simulink model "wheelControl"  (R2015a)
settings: Solver=ode45  StartTime=0.0  StopTime=10.0  RelTol=1e-3
libraries: simulink x2
settings Model: Creator=julig  LastModifiedBy=julig

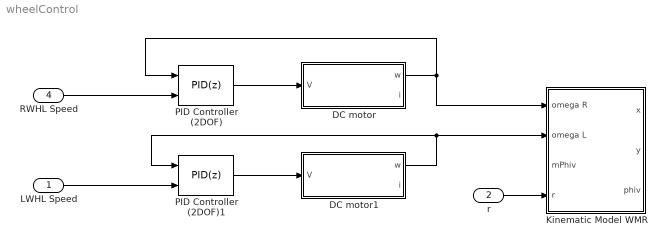
== system wheelControl ==
  "LWHL Speed " : Inport
  r : Inport  Port=2
  "RWHL Speed " : Inport  Port=4
  DC motor : Subsystem  mask(DC Motor){L=0.1, Kphi=0.3, J=0.1, b=0.01, R=2}
      mask help:
      | Takes the DC voltage as input, and outputs angular velocity (w) and current (i)
      | L => windings inductance		Kphi => emf constant
      | J => loads moment of inertial		b => viscous friction
      | R => windings resistance
      mask Display:
      | port_label('input', 1, 'V')
      | port_label('output', 2, 'i')
      | port_label('output', 1, 'w')
      | disp('DC Motor')
  DC motor1 : Subsystem  mask(DC Motor){L=0.1, Kphi=0.3, J=0.1, b=0.01, R=2}
      mask help:
      | Takes the DC voltage as input, and outputs angular velocity (w) and current (i)
      | L => windings inductance		Kphi => emf constant
      | J => loads moment of inertial		b => viscous friction
      | R => windings resistance
      mask Display:
      | port_label('input', 1, 'V')
      | port_label('output', 2, 'i')
      | port_label('output', 1, 'w')
      | disp('DC Motor')
  Kinematic Model WMR : Subsystem
  PID Controller (2DOF) : simulink/Continuous/PID Controller (2DOF)  Controller=PID  TimeDomain=Discrete-time  SampleTime=-1  IntegratorMethod=Forward Euler  FilterMethod=Forward Euler  Form=Parallel  UseFilter=on  ControllerParametersSource=internal  P=1  I=1  D=0  N=100  b=1  c=1  InitialConditionSource=internal  InitialConditionForIntegrator=0  InitialConditionForFilter=0  ExternalReset=none  LimitOutput=off  UpperSaturationLimit=inf  LowerSaturationLimit=-inf  LinearizeAsGain=on  AntiWindupMode=none  Kb=1  TrackingMode=off  Kt=1  PParamMin=[]  PParamMax=[]  IParamMin=[]  IParamMax=[]  DParamMin=[]  DParamMax=[]  NParamMin=[]  NParamMax=[]  bParamMin=[]  bParamMax=[]  cParamMin=[]  cParamMax=[]  KbParamMin=[]  KbParamMax=[]  KtParamMin=[]  KtParamMax=[]  POutMin=[]  POutMax=[]  IOutMin=[]  IOutMax=[]  DOutMin=[]  DOutMax=[]  NOutMin=[]  NOutMax=[]  bOutMin=[]  bOutMax=[]  cOutMin=[]  cOutMax=[]  KbOutMin=[]  KbOutMax=[]  KtOutMin=[]  KtOutMax=[]  IntegratorOutMin=[]  IntegratorOutMax=[]  FilterOutMin=[]  FilterOutMax=[]  SumOutMin=[]  SumOutMax=[]  Sum1OutMin=[]  Sum1OutMax=[]  Sum2OutMin=[]  Sum2OutMax=[]  Sum3OutMin=[]  Sum3OutMax=[]  SumI1OutMin=[]  SumI1OutMax=[]  SumI2OutMin=[]  SumI2OutMax=[]  SumI3OutMin=[]  SumI3OutMax=[]  SumDOutMin=[]  SumDOutMax=[]  SaturationOutMin=[]  SaturationOutMax=[]  IntegratorContinuousStateAttributes=''  IntegratorStateMustResolveToSignalObject=off  IntegratorRTWStateStorageClass=Auto  FilterContinuousStateAttributes=''  FilterStateMustResolveToSignalObject=off  FilterRTWStateStorageClass=Auto  DifferentiatorICPrevScaledInput=0  DifferentiatorOutMin=[]  DifferentiatorOutMax=[]
  PID Controller (2DOF)1 : simulink/Continuous/PID Controller (2DOF)  Controller=PID  TimeDomain=Discrete-time  SampleTime=-1  IntegratorMethod=Forward Euler  FilterMethod=Forward Euler  Form=Parallel  UseFilter=on  ControllerParametersSource=internal  P=1  I=1  D=0  N=100  b=1  c=1  InitialConditionSource=internal  InitialConditionForIntegrator=0  InitialConditionForFilter=0  ExternalReset=none  LimitOutput=off  UpperSaturationLimit=inf  LowerSaturationLimit=-inf  LinearizeAsGain=on  AntiWindupMode=none  Kb=1  TrackingMode=off  Kt=1  PParamMin=[]  PParamMax=[]  IParamMin=[]  IParamMax=[]  DParamMin=[]  DParamMax=[]  NParamMin=[]  NParamMax=[]  bParamMin=[]  bParamMax=[]  cParamMin=[]  cParamMax=[]  KbParamMin=[]  KbParamMax=[]  KtParamMin=[]  KtParamMax=[]  POutMin=[]  POutMax=[]  IOutMin=[]  IOutMax=[]  DOutMin=[]  DOutMax=[]  NOutMin=[]  NOutMax=[]  bOutMin=[]  bOutMax=[]  cOutMin=[]  cOutMax=[]  KbOutMin=[]  KbOutMax=[]  KtOutMin=[]  KtOutMax=[]  IntegratorOutMin=[]  IntegratorOutMax=[]  FilterOutMin=[]  FilterOutMax=[]  SumOutMin=[]  SumOutMax=[]  Sum1OutMin=[]  Sum1OutMax=[]  Sum2OutMin=[]  Sum2OutMax=[]  Sum3OutMin=[]  Sum3OutMax=[]  SumI1OutMin=[]  SumI1OutMax=[]  SumI2OutMin=[]  SumI2OutMax=[]  SumI3OutMin=[]  SumI3OutMax=[]  SumDOutMin=[]  SumDOutMax=[]  SaturationOutMin=[]  SaturationOutMax=[]  IntegratorContinuousStateAttributes=''  IntegratorStateMustResolveToSignalObject=off  IntegratorRTWStateStorageClass=Auto  FilterContinuousStateAttributes=''  FilterStateMustResolveToSignalObject=off  FilterRTWStateStorageClass=Auto  DifferentiatorICPrevScaledInput=0  DifferentiatorOutMin=[]  DifferentiatorOutMax=[]
  wires:
  "RWHL Speed "/1 -> PID Controller (2DOF)/2
  PID Controller (2DOF)/1 -> DC motor/1(V)
  DC motor/1(w) -> PID Controller (2DOF)/1, Kinematic Model WMR/1(omega R)
  DC motor1/1(w) -> PID Controller (2DOF)1/1, Kinematic Model WMR/2("omega L ")
  PID Controller (2DOF)1/1 -> DC motor1/1(V)
  "LWHL Speed "/1 -> PID Controller (2DOF)1/2
  r/1 -> Kinematic Model WMR/4(r)

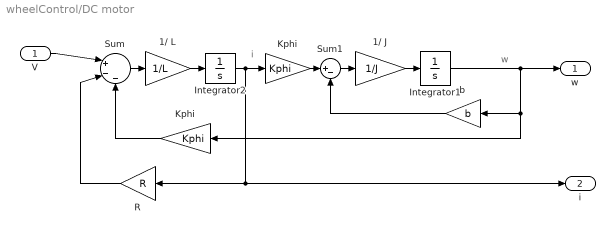
== system wheelControl/DC motor ==
  note: w
  note: i
  V : Inport
  1/ J : Gain  Gain=1/J
  1/ L : Gain  Gain=1/L
  Integrator1 : Integrator
  Integrator2 : Integrator
  Kphi : Gain  Gain=Kphi
  "Kphi " : Gain  Gain=Kphi
  R : Gain  Gain=R
  Sum : Sum  Inputs=|+--
  Sum1 : Sum  Inputs=|+-
  b : Gain  Gain=b
  w : Outport
  i : Outport  Port=2
  wires:
  R/1 -> Sum/2
  "Kphi "/1 -> Sum/3
  b/1 -> Sum1/2
  Integrator1/1 -> w/1, b/1, "Kphi "/1
  1/ J/1 -> Integrator1/1
  Sum1/1 -> 1/ J/1
  Kphi/1 -> Sum1/1
  Integrator2/1 -> i/1, R/1, Kphi/1
  1/ L/1 -> Integrator2/1
  Sum/1 -> 1/ L/1
  V/1 -> Sum/1

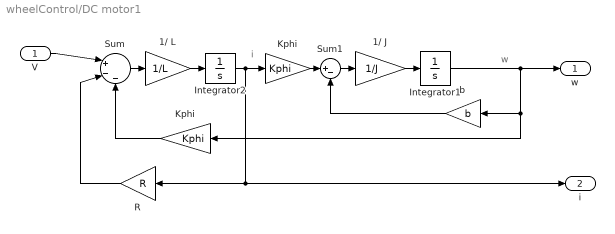
== system wheelControl/DC motor1 ==
  note: w
  note: i
  V : Inport
  1/ J : Gain  Gain=1/J
  1/ L : Gain  Gain=1/L
  Integrator1 : Integrator
  Integrator2 : Integrator
  Kphi : Gain  Gain=Kphi
  "Kphi " : Gain  Gain=Kphi
  R : Gain  Gain=R
  Sum : Sum  Inputs=|+--
  Sum1 : Sum  Inputs=|+-
  b : Gain  Gain=b
  w : Outport
  i : Outport  Port=2
  wires:
  R/1 -> Sum/2
  "Kphi "/1 -> Sum/3
  b/1 -> Sum1/2
  Integrator1/1 -> w/1, b/1, "Kphi "/1
  1/ J/1 -> Integrator1/1
  Sum1/1 -> 1/ J/1
  Kphi/1 -> Sum1/1
  Integrator2/1 -> i/1, R/1, Kphi/1
  1/ L/1 -> Integrator2/1
  Sum/1 -> 1/ L/1
  V/1 -> Sum/1

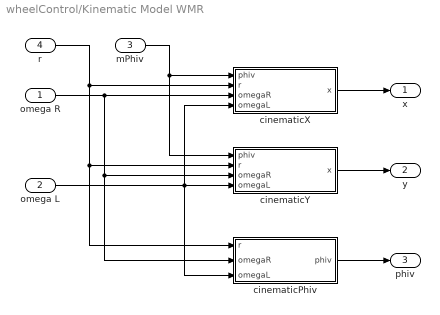
== system wheelControl/Kinematic Model WMR ==
  omega R : Inport
  "omega L " : Inport  Port=2
  mPhiv : Inport  Port=3
  r : Inport  Port=4
  cinematicPhiv : Subsystem
  cinematicX : Subsystem
  cinematicY : Subsystem
  x : Outport
  y : Outport  Port=2
  phiv : Outport  Port=3
  wires:
  omega R/1 -> cinematicPhiv/2(omegaR), cinematicY/3(omegaR), cinematicX/3(omegaR)
  "omega L "/1 -> cinematicY/4(omegaL), cinematicPhiv/3(omegaL), cinematicX/4(omegaL)
  cinematicX/1(x) -> x/1
  mPhiv/1 -> cinematicY/1(phiv), cinematicX/1(phiv)
  r/1 -> cinematicX/2(r), cinematicY/2(r), cinematicPhiv/1(r)
  cinematicY/1(x) -> y/1
  cinematicPhiv/1(phiv) -> phiv/1

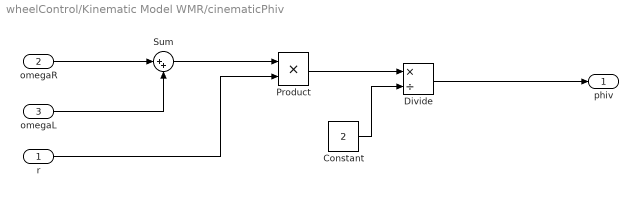
== system wheelControl/Kinematic Model WMR/cinematicPhiv ==
  r : Inport
  omegaR : Inport  Port=2
  omegaL : Inport  Port=3
  Constant : Constant  Value=2
  Divide : Product  Inputs=*/
  Product : Product
  Sum : Sum  Inputs=|++
  phiv : Outport
  wires:
  omegaR/1 -> Sum/1
  omegaL/1 -> Sum/2
  Sum/1 -> Product/1
  r/1 -> Product/2
  Product/1 -> Divide/1
  Constant/1 -> Divide/2
  Divide/1 -> phiv/1

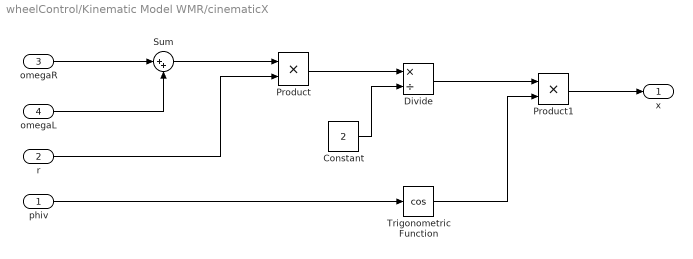
== system wheelControl/Kinematic Model WMR/cinematicX ==
  phiv : Inport
  r : Inport  Port=2
  omegaR : Inport  Port=3
  omegaL : Inport  Port=4
  Constant : Constant  Value=2
  Divide : Product  Inputs=*/
  Product : Product
  Product1 : Product
  Sum : Sum  Inputs=|++
  Trigonometric Function : Trigonometry  Operator=cos
  x : Outport
  wires:
  omegaR/1 -> Sum/1
  omegaL/1 -> Sum/2
  Sum/1 -> Product/1
  r/1 -> Product/2
  Product/1 -> Divide/1
  Constant/1 -> Divide/2
  Divide/1 -> Product1/1
  phiv/1 -> Trigonometric Function/1
  Trigonometric Function/1 -> Product1/2
  Product1/1 -> x/1

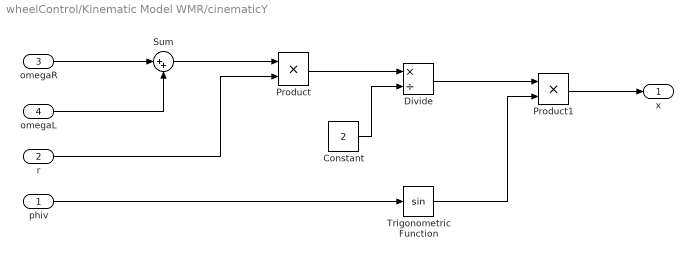
== system wheelControl/Kinematic Model WMR/cinematicY ==
  phiv : Inport
  r : Inport  Port=2
  omegaR : Inport  Port=3
  omegaL : Inport  Port=4
  Constant : Constant  Value=2
  Divide : Product  Inputs=*/
  Product : Product
  Product1 : Product
  Sum : Sum  Inputs=|++
  Trigonometric Function : Trigonometry
  x : Outport
  wires:
  omegaR/1 -> Sum/1
  omegaL/1 -> Sum/2
  Sum/1 -> Product/1
  r/1 -> Product/2
  Product/1 -> Divide/1
  Constant/1 -> Divide/2
  Divide/1 -> Product1/1
  phiv/1 -> Trigonometric Function/1
  Trigonometric Function/1 -> Product1/2
  Product1/1 -> x/1
